simulink model "IF_Flux_Romberg"  (R2022a)
settings: Solver=FixedStepDiscrete  StartTime=0.0  StopTime=3  FixedStep=0.000001  RelTol=1e-4  EnableMultiTasking=on
InitFcn:
  | Ld=5.25e-3;
  | Lq=12e-3;
  | R=0.958;
  | f=0.1827;
model workspace (MAT data in the model file):
  f = Simulink.Signal
  f.DataType = 'single'
  f.Dimensions = 1
  f.DimensionsMode = 'auto'
  f.Complexity = 'real'
  f.SampleTime = -1
  f.SamplingMode = 'auto'
  f.InitialValue = '0.1827'
values from neighbouring files (symbols this model uses):
  ki_c = 1476    [initialize.m]
  ki_pll = 900    [initialize.m]
  ki_sp = 0.5    [initialize.m]
  kp_c = 3.44    [initialize.m]
  kp_pll = 60    [initialize.m]
  kp_sp = 0.01    [initialize.m]
  L = 0.0014    [initialize.m]
  L1 = -5500    [initialize.m]
  L2 = 68500    [initialize.m]
  Rs = 0.6    [initialize.m]
  Ts = 0.0001    [initialize.m]
undefined symbols (not defined in the file or in its folder): DiscIntNeverNeededParam
libraries: slpidlib x6, mcbcontrolslib x5, eeGeneralControl x3, simulink x2, spsDCVoltageSourceLib x1, spsPermanentMagnetSynchronousMachineLib x1, spsUniversalBridgeLib x1, spspowerguiLib x1
settings Model: Creator=张豪  LastModifiedBy=EE
settings SolverCC: AutoInsertRateTranBlk=on
settings OptimizationCC: DefaultParameterBehavior=Inlined  UseDivisionForNetSlopeComputation=on  GainParamInheritBuiltInType=on  UseFloatMulNetSlope=on  InlineInvariantSignals=on  PassReuseOutputArgsAs=Individual arguments  ZeroExternalMemoryAtStartup=off  ZeroInternalMemoryAtStartup=off  NoFixptDivByZeroProtection=on  EfficientFloat2IntCast=on  LifeSpan=1  OptimizeBlockOrder=speed  DifferentSizesBufferReuse=on  EfficientTunableParamExpr=on
settings DebuggingCC: ParameterTunabilityLossMsg=error  UnconnectedInputMsg=warning  UnconnectedOutputMsg=warning  UnconnectedLineMsg=warning
settings HardwareCC: ProdLongLongMode=on
settings SFSimCC: MATLABDynamicMemAlloc=off
settings RTWCC: SystemTargetFile=ert.tlc  GenCodeOnly=on  TemplateMakefile=ert_default_tmf  DLArmComputeVersion=19.05
settings CodeAppCC: ForceParamTrailComments=on  IgnoreCustomStorageClasses=off  OperatorAnnotations=on  SimulinkDataObjDesc=on  SFDataObjDesc=on  CustomSymbolStrGlobalVar=rt$N$M  CustomSymbolStrType=$N$M  CustomSymbolStrFcn=$N$M$F  CustomSymbolStrMacro=$N$M  InsertBlockDesc=on
settings ERTTargetCC: TargetLangStandard=C99 (ISO)  GenerateSampleERTMain=on  IncludeMdlTerminateFcn=off  CombineSignalStateStructs=on  SupportComplex=off  SupportNonInlinedSFcns=on  InlinedParameterPlacement=NonHierarchical  ERTCustomFileTemplate=example_file_process.tlc  ERTFilePackagingFormat=CompactWithDataFile

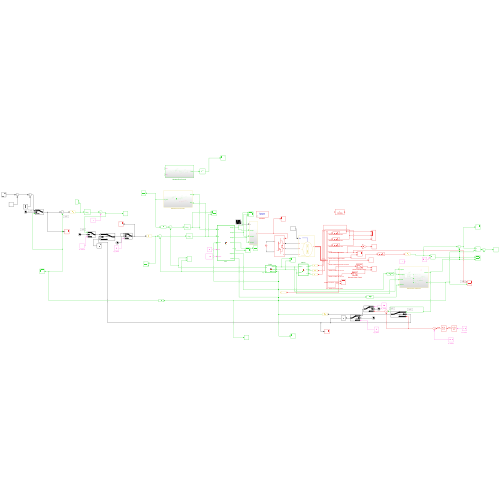
[thumbnail: Simulink's stored preview of the top-level diagram]
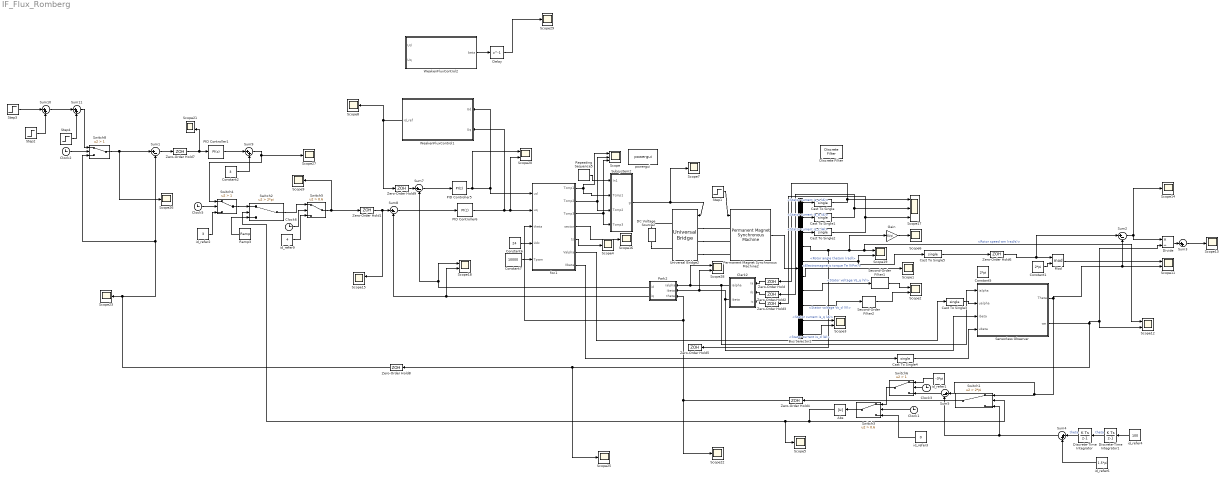
== system IF_Flux_Romberg ==
  Abs : Abs  SaturateOnIntegerOverflow=off
  Bus Selector2 : BusSelector  OutputSignals=Stator current is_a (A),Stator current is_b (A),Stator current is_c (A),Rotor speed wm (rad/s),Rotor angle thetam (rad),Electromagnetic torque Te (N*m),Stator voltage Vs_q (V),Stator voltage Vs_d (V),Stator current is_q (A),Stator current is_d (A)
  Cast To Single{,1..5} (6 alike) : DataTypeConversion  OutDataTypeStr=single  SaturateOnIntegerOverflow=off  RndMeth=Floor
  Clark2 : MATLAB Function  TreatAsAtomicUnit=on
  Clock{1..3,5..6} (5 alike) : Clock
  Constant1 : Constant  Value=2*pi  OutDataTypeStr=single
  Constant2 : Constant  Value=3
  Constant5 : Constant  Value=2*pi  OutDataTypeStr=single
  Constant6 : Constant  Value=24
  Constant7 : Constant  Value=10000  OutDataTypeStr=single
  DC Voltage Source2 : spsDCVoltageSourceLib/DC Voltage Source  Amplitude=24  Measurements=None
  Delay : Delay  DelayLength=1  InitialCondition=0
  Discrete Filter : DiscreteFilter  FilterStructure=Direct form I
  Discrete-Time Integrator : DiscreteIntegrator  SampleTime=-1  ICPrevOutput=DiscIntNeverNeededParam  ICPrevScaledInput=DiscIntNeverNeededParam
  Discrete-Time Integrator1 : DiscreteIntegrator  SampleTime=-1  ICPrevOutput=DiscIntNeverNeededParam  ICPrevScaledInput=DiscIntNeverNeededParam
  Divide : Product  Inputs=*/
  Gain : Gain  Gain=30/pi
  Mod : Math  Operator=mod
  PID Controller1 : slpidlib/PID Controller  Controller=PI  Form=Parallel  TimeDomain=Discrete-time  UseExternalTs=off  SampleTime=1e-4  IntegratorMethod=Forward Euler  FilterMethod=Forward Euler  ControllerParametersSource=internal  P=kp_sp  I=ki_sp  UseKiTs=off  D=0  N=100  UseFilter=on  TunerSelectOption=Transfer Function Based (PID Tuner App)  InitialConditionSource=internal  InitialConditionForIntegrator=0  InitialConditionForFilter=0  DifferentiatorICPrevScaledInput=0  ExternalReset=none  TrackingMode=off  Kt=1  LimitOutput=off  SatLimitsSource=internal  UpperSaturationLimit=7  LowerSaturationLimit=-7  LinearizeAsGain=on  AntiWindupMode=none  Kb=1  POutMin=[]  POutMax=[]  IOutMin=[]  IOutMax=[]  DOutMin=[]  DOutMax=[]  NOutMin=[]  NOutMax=[]  SumOutMin=[]  SumOutMax=[]  SaturationOutMin=[]  SaturationOutMax=[]  PParamMin=[]  PParamMax=[]  IParamMin=[]  IParamMax=[]  DParamMin=[]  DParamMax=[]  NParamMin=[]  NParamMax=[]  KbParamMin=[]  KbParamMax=[]  KtParamMin=[]  KtParamMax=[]  KbOutMin=[]  KbOutMax=[]  KtOutMin=[]  KtOutMax=[]  IntegratorOutMin=[]  IntegratorOutMax=[]  FilterOutMin=[]  FilterOutMax=[]  SumI1OutMin=[]  SumI1OutMax=[]  SumI2OutMin=[]  SumI2OutMax=[]  SumI3OutMin=[]  SumI3OutMax=[]  SumI4OutMin=[]  SumI4OutMax=[]  SumDOutMin=[]  SumDOutMax=[]  DifferentiatorOutMin=[]  DifferentiatorOutMax=[]  FilterDiffOutCoefMin=[]  FilterDiffOutCoefMax=[]  ReciprocalOutMin=[]  ReciprocalOutMax=[]  SumDenOutMin=[]  SumDenOutMax=[]  SumNumOutMin=[]  SumNumOutMax=[]  DivideOutMin=[]  DivideOutMax=[]  UdiffTsProdOutMin=[]  UdiffTsProdOutMax=[]  NTsProdOutMin=[]  NTsProdOutMax=[]  UintegralTsProdOutMin=[]  UintegralTsProdOutMax=[]  UngainTsProdOutMin=[]  UngainTsProdOutMax=[]  IntegratorContinuousStateAttributes=''  IntegratorStateMustResolveToSignalObject=off  IntegratorRTWStateStorageClass=Auto  FilterContinuousStateAttributes=''  FilterStateMustResolveToSignalObject=off  FilterRTWStateStorageClass=Auto  ParallelPVariant=InternalParameters  IdealPVariant=Disabled  IVariant=InternalParameters  DVariant=Disabled  IntegratorVariant=Discrete  SatVariant=Disabled  AWVariant=Passthrough  PCopyVariant=Disabled  TRVariant=Disabled  FdbkBlocksVariant=Forward  IdealPFdbkVariant=Disabled  SatFdbkVariant=Disabled  DerivativeFilterVariant=Disabled  NVariant=Disabled  NCopyVariant=Disabled_SignalSpec  FilterICVariant=Disabled  IntegratorICVariant=InternalICs  ExternalResetVariant=Disabled  TRSumVariant=Passthrough  SumFdbkVariant=Disabled  SumVariant=Sum_PI  TsampFilterVariant=InternalTs  TsampNgainVariant=Passthrough  TsampIntegralVariant=Passthrough  ExternalSaturationOutDataTypeStr=Inherit: Same as second input  aMode=0
  PID Controller5 : slpidlib/PID Controller  Controller=PI  Form=Parallel  TimeDomain=Discrete-time  UseExternalTs=off  SampleTime=1e-4  IntegratorMethod=Forward Euler  FilterMethod=Forward Euler  ControllerParametersSource=internal  P=kp_c  I=ki_c  UseKiTs=off  D=0  N=100  UseFilter=on  TunerSelectOption=Transfer Function Based (PID Tuner App)  InitialConditionSource=internal  InitialConditionForIntegrator=0  InitialConditionForFilter=0  DifferentiatorICPrevScaledInput=0  ExternalReset=none  TrackingMode=off  Kt=1  LimitOutput=off  SatLimitsSource=internal  UpperSaturationLimit=13  LowerSaturationLimit=-10  LinearizeAsGain=on  AntiWindupMode=none  Kb=1  POutMin=[]  POutMax=[]  IOutMin=[]  IOutMax=[]  DOutMin=[]  DOutMax=[]  NOutMin=[]  NOutMax=[]  SumOutMin=[]  SumOutMax=[]  SaturationOutMin=[]  SaturationOutMax=[]  PParamMin=[]  PParamMax=[]  IParamMin=[]  IParamMax=[]  DParamMin=[]  DParamMax=[]  NParamMin=[]  NParamMax=[]  KbParamMin=[]  KbParamMax=[]  KtParamMin=[]  KtParamMax=[]  KbOutMin=[]  KbOutMax=[]  KtOutMin=[]  KtOutMax=[]  IntegratorOutMin=[]  IntegratorOutMax=[]  FilterOutMin=[]  FilterOutMax=[]  SumI1OutMin=[]  SumI1OutMax=[]  SumI2OutMin=[]  SumI2OutMax=[]  SumI3OutMin=[]  SumI3OutMax=[]  SumI4OutMin=[]  SumI4OutMax=[]  SumDOutMin=[]  SumDOutMax=[]  DifferentiatorOutMin=[]  DifferentiatorOutMax=[]  FilterDiffOutCoefMin=[]  FilterDiffOutCoefMax=[]  ReciprocalOutMin=[]  ReciprocalOutMax=[]  SumDenOutMin=[]  SumDenOutMax=[]  SumNumOutMin=[]  SumNumOutMax=[]  DivideOutMin=[]  DivideOutMax=[]  UdiffTsProdOutMin=[]  UdiffTsProdOutMax=[]  NTsProdOutMin=[]  NTsProdOutMax=[]  UintegralTsProdOutMin=[]  UintegralTsProdOutMax=[]  UngainTsProdOutMin=[]  UngainTsProdOutMax=[]  IntegratorContinuousStateAttributes=''  IntegratorStateMustResolveToSignalObject=off  IntegratorRTWStateStorageClass=Auto  FilterContinuousStateAttributes=''  FilterStateMustResolveToSignalObject=off  FilterRTWStateStorageClass=Auto  ParallelPVariant=InternalParameters  IdealPVariant=Disabled  IVariant=InternalParameters  DVariant=Disabled  IntegratorVariant=Discrete  SatVariant=Disabled  AWVariant=Passthrough  PCopyVariant=Disabled  TRVariant=Disabled  FdbkBlocksVariant=Forward  IdealPFdbkVariant=Disabled  SatFdbkVariant=Disabled  DerivativeFilterVariant=Disabled  NVariant=Disabled  NCopyVariant=Disabled_SignalSpec  FilterICVariant=Disabled  IntegratorICVariant=InternalICs  ExternalResetVariant=Disabled  TRSumVariant=Passthrough  SumFdbkVariant=Disabled  SumVariant=Sum_PI  TsampFilterVariant=InternalTs  TsampNgainVariant=Passthrough  TsampIntegralVariant=Passthrough  ExternalSaturationOutDataTypeStr=Inherit: Same as second input  aMode=0
  PID Controller6 : slpidlib/PID Controller  Controller=PI  Form=Parallel  TimeDomain=Discrete-time  UseExternalTs=off  SampleTime=1e-4  IntegratorMethod=Forward Euler  FilterMethod=Forward Euler  ControllerParametersSource=internal  P=kp_c  I=ki_c  UseKiTs=off  D=0  N=100  UseFilter=on  TunerSelectOption=Transfer Function Based (PID Tuner App)  InitialConditionSource=internal  InitialConditionForIntegrator=0  InitialConditionForFilter=0  DifferentiatorICPrevScaledInput=0  ExternalReset=none  TrackingMode=off  Kt=1  LimitOutput=off  SatLimitsSource=internal  UpperSaturationLimit=14  LowerSaturationLimit=0  LinearizeAsGain=on  AntiWindupMode=none  Kb=1  POutMin=[]  POutMax=[]  IOutMin=[]  IOutMax=[]  DOutMin=[]  DOutMax=[]  NOutMin=[]  NOutMax=[]  SumOutMin=[]  SumOutMax=[]  SaturationOutMin=[]  SaturationOutMax=[]  PParamMin=[]  PParamMax=[]  IParamMin=[]  IParamMax=[]  DParamMin=[]  DParamMax=[]  NParamMin=[]  NParamMax=[]  KbParamMin=[]  KbParamMax=[]  KtParamMin=[]  KtParamMax=[]  KbOutMin=[]  KbOutMax=[]  KtOutMin=[]  KtOutMax=[]  IntegratorOutMin=[]  IntegratorOutMax=[]  FilterOutMin=[]  FilterOutMax=[]  SumI1OutMin=[]  SumI1OutMax=[]  SumI2OutMin=[]  SumI2OutMax=[]  SumI3OutMin=[]  SumI3OutMax=[]  SumI4OutMin=[]  SumI4OutMax=[]  SumDOutMin=[]  SumDOutMax=[]  DifferentiatorOutMin=[]  DifferentiatorOutMax=[]  FilterDiffOutCoefMin=[]  FilterDiffOutCoefMax=[]  ReciprocalOutMin=[]  ReciprocalOutMax=[]  SumDenOutMin=[]  SumDenOutMax=[]  SumNumOutMin=[]  SumNumOutMax=[]  DivideOutMin=[]  DivideOutMax=[]  UdiffTsProdOutMin=[]  UdiffTsProdOutMax=[]  NTsProdOutMin=[]  NTsProdOutMax=[]  UintegralTsProdOutMin=[]  UintegralTsProdOutMax=[]  UngainTsProdOutMin=[]  UngainTsProdOutMax=[]  IntegratorContinuousStateAttributes=''  IntegratorStateMustResolveToSignalObject=off  IntegratorRTWStateStorageClass=Auto  FilterContinuousStateAttributes=''  FilterStateMustResolveToSignalObject=off  FilterRTWStateStorageClass=Auto  ParallelPVariant=InternalParameters  IdealPVariant=Disabled  IVariant=InternalParameters  DVariant=Disabled  IntegratorVariant=Discrete  SatVariant=Disabled  AWVariant=Passthrough  PCopyVariant=Disabled  TRVariant=Disabled  FdbkBlocksVariant=Forward  IdealPFdbkVariant=Disabled  SatFdbkVariant=Disabled  DerivativeFilterVariant=Disabled  NVariant=Disabled  NCopyVariant=Disabled_SignalSpec  FilterICVariant=Disabled  IntegratorICVariant=InternalICs  ExternalResetVariant=Disabled  TRSumVariant=Passthrough  SumFdbkVariant=Disabled  SumVariant=Sum_PI  TsampFilterVariant=InternalTs  TsampNgainVariant=Passthrough  TsampIntegralVariant=Passthrough  ExternalSaturationOutDataTypeStr=Inherit: Same as second input  aMode=0
  Park2 : MATLAB Function  TreatAsAtomicUnit=on
  Permanent Magnet Synchronous Machine2 : spsPermanentMagnetSynchronousMachineLib/Permanent Magnet Synchronous Machine  NbPhases=3  FluxDistribution=Sinusoidal  RotorType=Round  MechanicalLoad=Torque Tm  PresetModel=No  ShowDetailedParameters=on  MeasurementBus=off  Resistance=0.6  Inductance=8.5e-3  dqInductances=[5.25e-3 12e-3]  La=1.4e-3  MachineConstant=Flux linkage established by magnets (V.s)  Flux=0.034182  VoltageCst=6.1999  TorqueCst=0.051273  Flat=120  Mechanical=[1.1e-5 0.001 1 0.02]  PolePairs=4  InitialConditions=[0,0, 0,0]  InitialConditions5ph=[0 0 0 0 0 0]  RefAngle=Aligned with phase A axis (original Park)  IterativeDiscreteModel=Trapezoidal non iterative  TsBlock=-1  TsPowergui=0
  Ramp3 : simulink/Sources/Ramp  slope=-10  start=0.6  InitialOutput=4
  Repeating Sequence5 : simulink/Sources/Repeating Sequence  rep_seq_t=[0 0.00005 0.0001]  rep_seq_y=[0 5000 0]
  Scope : Scope  NumInputPorts=3
  Scope{1,4..9,13..14,16,22..23,25..27,29} (16 alike) : Scope
  Scope{2..3,11..12,15,18..21,28} (10 alike) : Scope  NumInputPorts=2
  Scope17 : Scope  NumInputPorts=3
  Second-Order Filter1 : eeGeneralControl/Second-Order Filter  FilterType=Low-pass  fn=100  Zeta=1  Ts=-1  A0=0  Ph0=0  f0=0  b0=0
      settings: SourceProductBaseCode=PS
  Second-Order Filter2 : eeGeneralControl/Second-Order Filter  FilterType=Low-pass  fn=100  Zeta=1  Ts=-1  A0=0  Ph0=0  f0=0  b0=0
      settings: SourceProductBaseCode=PS
  Sensorless Observer : Subsystem
  Step1 : Step  Time=0.6  Before=0.05  After=0.05  SampleTime=0
  Step2 : Step  Time=2  After=80  SampleTime=0
  Step3 : Step  Time=1.5  Before=150  After=200  SampleTime=0
  Step4 : Step  Time=2.5  After=-100  SampleTime=0
  Subsystem2 : Subsystem
  Sum{1..2,5,7..8} (5 alike) : Sum  Inputs=|+-
  Sum{3..4,9..11} (5 alike) : Sum  Inputs=|++
  Switch1 : Switch  Criteria=u2 > Threshold  Threshold=2*pi  SaturateOnIntegerOverflow=off  InputSameDT=off
  Switch2 : Switch  Criteria=u2 > Threshold  Threshold=2*pi  SaturateOnIntegerOverflow=off  InputSameDT=off
  Switch3 : Switch  Criteria=u2 > Threshold  Threshold=0.6  SaturateOnIntegerOverflow=off  InputSameDT=off
  Switch4 : Switch  Criteria=u2 > Threshold  Threshold=1  SaturateOnIntegerOverflow=off  InputSameDT=off
  Switch5 : Switch  Criteria=u2 > Threshold  Threshold=0.6  SaturateOnIntegerOverflow=off  InputSameDT=off
  Switch6 : Switch  Criteria=u2 > Threshold  Threshold=1  SaturateOnIntegerOverflow=off  InputSameDT=off
  Switch8 : Switch  Criteria=u2 > Threshold  Threshold=1  SaturateOnIntegerOverflow=off  InputSameDT=off
  Universal Bridge2 : spsUniversalBridgeLib/Universal Bridge  Arms=3  SnubberResistance=1e5  SnubberCapacitance=inf  Device=IGBT / Diodes  Ron=1e-3  Lon=0  ForwardVoltages="[  0  0  ]"  ForwardVoltage=0  GTOparameters=[ 10e-6 , 20e-6 ]  IGBTparameters=[ 1e-6 , 2e-6 ]  Measurements=None  Measurements_2=None  converterType=Rectifier
  WeakenFluxControl1 : Subsystem
  WeakenFluxControl2 : Subsystem
  Zero-Order Hold{,1..9} (10 alike) : ZeroOrderHold  SampleTime=1e-4
  foc1 : MATLAB Function  TreatAsAtomicUnit=on
  id_refer1 : Constant  Value=-3*pi
  id_refer2 : Constant  Value=3
  id_refer3 : Constant  Value=0
  id_refer4 : Constant  Value=100
  id_refer6 : Constant  Value=1.5*pi
  id_refer9 : Constant  Value=4
  powergui : spspowerguiLib/powergui  Priority=1  SimulationMode=Discrete  SampleTime=1e-6  frequency=60  Iterations=50  frequencyindice=0  Pbase=100e6  ErrMax=1e-4  UnitsV=kV  UnitsW=MW  buscounter=0  FunctionMessages=off  echomessages=off  EnableUseOfTLC=off  CurrentSourceSwitches=off  DisableSnubberDevices=off  DisableRonSwitches=off  DisableVfSwitches=off  DisplayEquations=off  AutomaticDiscreteSolvers=off  SolverType=Tustin/Backward Euler (TBE)  Interpol=off  ExternalGateDelay=off  methode=off  Ts=100  x0status=blocks  SPID=on  SwTol=0  HookPort=off  NonlinearTolerance=1e-4  nMaxIteration=100  ContinueOnMaxIteration=off  RestoreLinks=warning  ResistiveCurrentMeasurement=off  Frange=[0:2:500]  Ylog=off  Xlog=on  ShowGrid=off  save=off  variable=ZData  structure=0  ZoomFFT=off  StartTime=0.0  cycles=1  DisplayStyle=1  fundamental=60  FreqAxis=off  MaxFrequency=1000  frequencyindicesteady=1  RmsSteady=1  display=off
  wires:
  Repeating Sequence5/1 -> Subsystem2/1(In1)
  Constant7/1 -> foc1/5(Tpwm)
  foc1/3(Tcmp3) -> Subsystem2/4(Tcmp3), Scope/3
  foc1/2(Tcmp2) -> Subsystem2/3(Tcmp2), Scope/2
  Constant6/1 -> foc1/4(Udc)
  foc1/1(Tcmp1) -> Subsystem2/2(Tcmp1), Scope/1
  foc1/4(sector) -> Scope16/1
  Subsystem2/1(g) -> Scope7/1, Universal Bridge2/1
  Permanent Magnet Synchronous Machine2/1 -> Bus Selector2/1
  Bus Selector2/1 -> Cast To Single/1  "<Stator current is_a (A)>"
  Bus Selector2/2 -> Cast To Single1/1  "<Stator current is_b (A)>"
  Bus Selector2/3 -> Cast To Single2/1  "<Stator current is_c (A)>"
  Bus Selector2/5 -> Scope19/2, Cast To Single5/1  "<Rotor angle thetam (rad)>"
  Bus Selector2/4 -> Scope12/1, Scope19/1, Gain/1, Zero-Order Hold5/1  "<Rotor speed wm (rad/s)>"
  Bus Selector2/6 -> Scope1/1  "<Electromagnetic torque Te (N*m)>"
  Bus Selector2/7 -> Second-Order Filter1/1  "<Stator voltage Vs_q (V)>"
  Bus Selector2/8 -> Second-Order Filter2/1  "<Stator voltage Vs_d (V)>"
  Second-Order Filter1/1 -> Scope2/1
  Second-Order Filter2/1 -> Scope2/2
  Bus Selector2/9 -> Scope3/1  "<Stator current is_q (A)>"
  Bus Selector2/10 -> Scope3/2  "<Stator current is_d (A)>"
  foc1/5(ts) -> Scope4/1
  Gain/1 -> Scope6/1
  Zero-Order Hold/1 -> Clark2/1(ia)
  Zero-Order Hold2/1 -> Clark2/2(ib)
  Zero-Order Hold3/1 -> Clark2/3(ic)
  Zero-Order Hold4/1 -> foc1/3(theta), Park2/3(theta), Scope22/1
  Sum8/1 -> PID Controller6/1
  Step1/1 -> Permanent Magnet Synchronous Machine2/1
  Cast To Single/1 -> Zero-Order Hold/1, Scope17/1
  Cast To Single1/1 -> Zero-Order Hold2/1, Scope17/2
  Cast To Single2/1 -> Zero-Order Hold3/1, Scope17/3
  foc1/6(Valpha) -> Cast To Single3/1
  foc1/7(Vbeta) -> Cast To Single4/1
  Cast To Single3/1 -> Sensorless Observer/2(ualpha)
  Cast To Single4/1 -> Sensorless Observer/4(ubeta)
  Cast To Single5/1 -> Zero-Order Hold6/1
  Constant1/1 -> Mod/2
  Zero-Order Hold6/1 -> Sum2/1, Mod/1
  Sum2/1 -> Divide/1, Scope14/1
  Divide/1 -> Sum3/1
  Sum3/1 -> Scope13/1
  Zero-Order Hold1/1 -> Scope15/1, Sum8/1
  Switch8/1 -> Sum1/1, Scope26/1
  Discrete-Time Integrator1/1 -> Discrete-Time Integrator/1  "theta"
  Discrete-Time Integrator/1 -> Sum4/1  "theta"
  id_refer4/1 -> Discrete-Time Integrator1/1
  id_refer6/1 -> Sum4/2
  id_refer9/1 -> Switch5/3
  Clock6/1 -> Switch5/2
  Sum7/1 -> PID Controller5/1
  Sum4/1 -> Sum5/2, Switch1/3
  Zero-Order Hold8/1 -> Switch8/3, Sum1/2, Scope23/1
  Ramp3/1 -> Switch2/3
  Switch2/1 -> Switch5/1
  Switch3/1 -> Abs/1
  id_refer3/1 -> Switch3/3
  Clock1/1 -> Switch3/2
  Zero-Order Hold7/1 -> Scope21/2, PID Controller1/1
  Clock2/1 -> Switch8/2
  Clock5/1 -> Switch4/2
  id_refer2/1 -> Switch4/3
  Sensorless Observer/1(Theta) -> Scope11/2, Sum2/2, Switch1/1, Sum5/1
  Abs/1 -> Scope5/1, Switch2/2, Switch1/2
  Zero-Order Hold9/1 -> Sum7/1
  Constant2/1 -> Sum9/2
  Sum1/1 -> Zero-Order Hold7/1
  PID Controller1/1 -> Sum9/1
  Sum9/1 -> Scope27/1, Switch4/1
  Step3/1 -> Sum10/1
  Switch4/1 -> Switch2/1
  Clark2/1(ialpha) -> Sensorless Observer/1(ialpha), Scope28/1, Park2/1(ialpha)
  Clark2/2(ibeta) -> Sensorless Observer/3(ibeta), Scope28/2, Park2/2(ibeta)
  Sensorless Observer/2(we) -> Divide/2, Scope12/2, Zero-Order Hold8/1, Scope25/1
  Step2/1 -> Sum10/2
  Sum10/1 -> Sum11/1
  Sum11/1 -> Switch8/1
  Step4/1 -> Sum11/2
  Mod/1 -> Scope11/1
  WeakenFluxControl1/1(id_ref) -> Scope8/1, Zero-Order Hold9/1
  Park2/2(iq) -> Scope18/2, Sum8/2
  Park2/1(id) -> Scope18/1, Sum7/2
  PID Controller6/1 -> foc1/2(uq), Scope20/2, WeakenFluxControl1/2(Uq)
  PID Controller5/1 -> WeakenFluxControl1/1(Ud), foc1/1(ud), Scope20/1
  Switch1/1 -> Zero-Order Hold4/1
  Sum5/1 -> Switch6/3
  Clock3/1 -> Switch6/2
  id_refer1/1 -> Switch6/1
  Switch6/1 -> Switch3/1
  Delay/1 -> Scope29/1
  WeakenFluxControl2/1(beta) -> Delay/1
  Switch5/1 -> Scope9/1, Zero-Order Hold1/1
  connections:
  DC Voltage Source2/LConn1 -- Universal Bridge2/RConn2
  DC Voltage Source2/RConn1 -- Universal Bridge2/RConn1
  Universal Bridge2/LConn1 -- Permanent Magnet Synchronous Machine2/LConn1
  Universal Bridge2/LConn3 -- Permanent Magnet Synchronous Machine2/LConn3
  Universal Bridge2/LConn2 -- Permanent Magnet Synchronous Machine2/LConn2

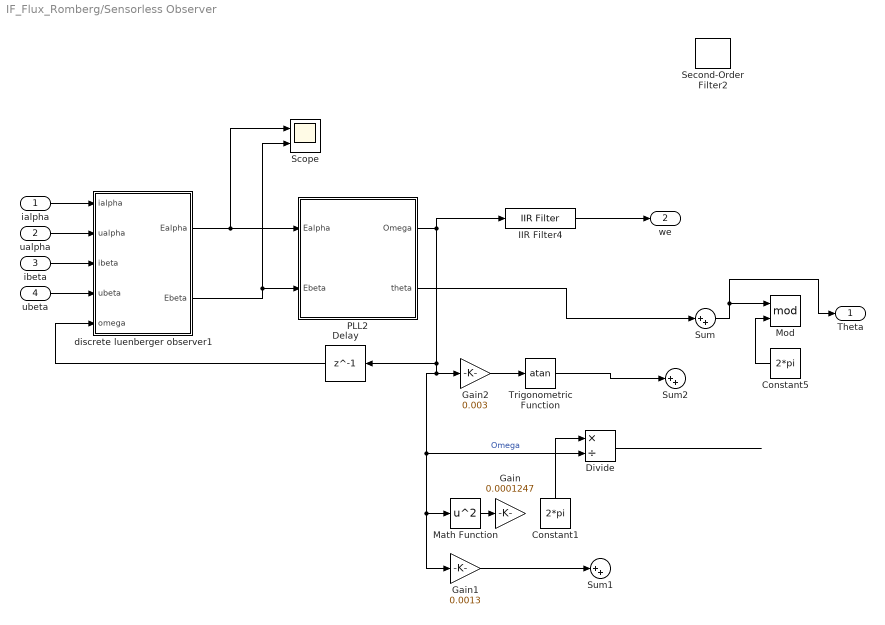
== system IF_Flux_Romberg/Sensorless Observer ==
  ialpha : Inport  OutDataTypeStr=single
  ualpha : Inport  Port=2  OutDataTypeStr=single
  ibeta : Inport  Port=3  OutDataTypeStr=single
  ubeta : Inport  Port=4  OutDataTypeStr=single
  Constant1 : Constant  Value=2*pi  OutDataTypeStr=single
  Constant5 : Constant  Value=2*pi  OutDataTypeStr=single
  Delay : Delay  DelayLength=1  InputProcessing=Columns as channels (frame based)
  Divide : Product  Inputs=*/
  Gain : Gain  Gain=0.0001247
  Gain1 : Gain  Gain=0.0013
  Gain2 : Gain  Gain=0.003
  IIR Filter4 : mcbcontrolslib/IIR Filter  VariantControl=Low Pass Filter  VariantSelect=Low-pass  Filter_constant=0.01  advancedSettings=on  Ts=1e-4  cutOff_freq=16.0763
      settings: SourceProductBaseCode=MT
  Math Function : Math  Operator=square
  Mod : Math  Operator=mod
  PLL2 : Subsystem
  Scope : Scope  NumInputPorts=2
  Second-Order Filter2 : eeGeneralControl/Second-Order Filter  FilterType=Low-pass  fn=100  Zeta=1  Ts=-1  A0=0  Ph0=0  f0=0  b0=0
      settings: SourceProductBaseCode=PS
  Sum : Sum  Inputs=|++
  Sum1 : Sum  Inputs=|++
  Sum2 : Sum  Inputs=|++
  Trigonometric Function : Trigonometry  Operator=atan
  discrete luenberger observer1 : Subsystem
  Theta : Outport
  we : Outport  Port=2
  wires:
  ubeta/1 -> discrete luenberger observer1/4(ubeta)
  ualpha/1 -> discrete luenberger observer1/2(ualpha)
  ibeta/1 -> discrete luenberger observer1/3(ibeta)
  ialpha/1 -> discrete luenberger observer1/1(ialpha)
  discrete luenberger observer1/1(Ealpha) -> Scope/1, PLL2/1(Ealpha)
  discrete luenberger observer1/2(Ebeta) -> Scope/2, PLL2/2(Ebeta)
  Constant5/1 -> Mod/2
  Delay/1 -> discrete luenberger observer1/5(omega)
  PLL2/2(theta) -> Sum/1
  Sum/1 -> Theta/1, Mod/1
  Math Function/1 -> Gain/1
  PLL2/1(Omega) -> IIR Filter4/1, Delay/1, Gain1/1, Math Function/1, Divide/2, Gain2/1  "Omega"
  Gain1/1 -> Sum1/1
  Constant1/1 -> Divide/1
  Gain2/1 -> Trigonometric Function/1
  Trigonometric Function/1 -> Sum2/1
  IIR Filter4/1 -> we/1
  Divide/1 -> ?

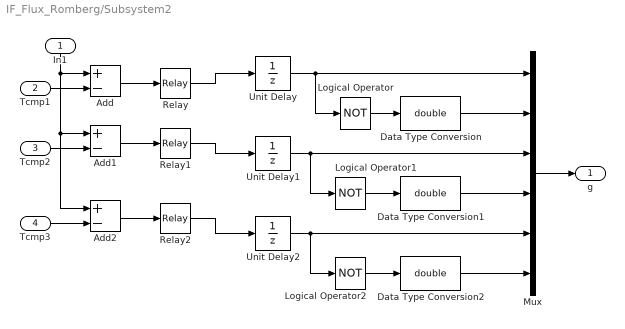
== system IF_Flux_Romberg/Subsystem2 ==
  In1 : Inport
  Tcmp1 : Inport  Port=2
  Tcmp2 : Inport  Port=3
  Tcmp3 : Inport  Port=4
  Add : Sum  Inputs=+-
  Add1 : Sum  Inputs=+-
  Add2 : Sum  Inputs=+-
  Data Type Conversion : DataTypeConversion  OutDataTypeStr=double  SaturateOnIntegerOverflow=off  RndMeth=Floor
  Data Type Conversion1 : DataTypeConversion  OutDataTypeStr=double  SaturateOnIntegerOverflow=off  RndMeth=Floor
  Data Type Conversion2 : DataTypeConversion  OutDataTypeStr=double  SaturateOnIntegerOverflow=off  RndMeth=Floor
  Logical Operator : Logic  Operator=NOT  AllPortsSameDT=off  OutDataTypeStr=boolean
  Logical Operator1 : Logic  Operator=NOT  AllPortsSameDT=off  OutDataTypeStr=boolean
  Logical Operator2 : Logic  Operator=NOT  AllPortsSameDT=off  OutDataTypeStr=boolean
  Mux : Mux  Inputs=6
  Relay : Relay  OffSwitchValue=-eps
  Relay1 : Relay  OffSwitchValue=-eps
  Relay2 : Relay  OffSwitchValue=-eps
  Unit Delay : UnitDelay  SampleTime=-1  HasFrameUpgradeWarning=on
  Unit Delay1 : UnitDelay  SampleTime=-1  HasFrameUpgradeWarning=on
  Unit Delay2 : UnitDelay  SampleTime=-1  HasFrameUpgradeWarning=on
  g : Outport  VectorParamsAs1DForOutWhenUnconnected=off
  wires:
  Tcmp3/1 -> Add2/2
  Tcmp2/1 -> Add1/2
  Tcmp1/1 -> Add/2
  Relay2/1 -> Unit Delay2/1
  Relay1/1 -> Unit Delay1/1
  Relay/1 -> Unit Delay/1
  Unit Delay2/1 -> Mux/5, Logical Operator2/1
  Unit Delay1/1 -> Mux/3, Logical Operator1/1
  Unit Delay/1 -> Logical Operator/1, Mux/1
  Mux/1 -> g/1
  Data Type Conversion/1 -> Mux/2
  Data Type Conversion1/1 -> Mux/4
  Data Type Conversion2/1 -> Mux/6
  Logical Operator2/1 -> Data Type Conversion2/1
  Logical Operator1/1 -> Data Type Conversion1/1
  Logical Operator/1 -> Data Type Conversion/1
  Add1/1 -> Relay1/1
  Add2/1 -> Relay2/1
  Add/1 -> Relay/1
  In1/1 -> Add/1, Add2/1, Add1/1

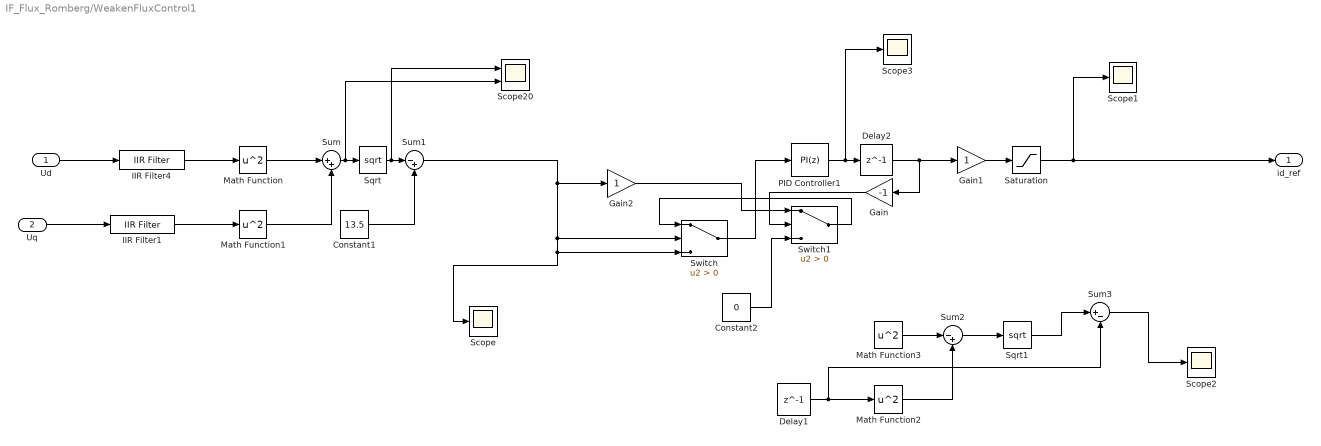
== system IF_Flux_Romberg/WeakenFluxControl1 ==
  Ud : Inport  OutDataTypeStr=double
  Uq : Inport  Port=2  OutDataTypeStr=double
  Constant1 : Constant  Value=13.5
  Constant2 : Constant  Value=0
  Delay1 : Delay  DelayLength=1  InitialCondition=0
  Delay2 : Delay  DelayLength=1  InitialCondition=0
  Gain : Gain  Gain=-1
  Gain1 : Gain
  Gain2 : Gain
  IIR Filter1 : mcbcontrolslib/IIR Filter  VariantControl=Low Pass Filter  VariantSelect=Low-pass  Filter_constant=0.05  advancedSettings=on  Ts=1e-4  cutOff_freq=83.7658
      settings: SourceProductBaseCode=MT
  IIR Filter4 : mcbcontrolslib/IIR Filter  VariantControl=Low Pass Filter  VariantSelect=Low-pass  Filter_constant=0.05  advancedSettings=on  Ts=1e-4  cutOff_freq=83.7658
      settings: SourceProductBaseCode=MT
  Math Function{,1..3} (4 alike) : Math  Operator=square
  PID Controller1 : slpidlib/PID Controller  Controller=PI  Form=Parallel  TimeDomain=Discrete-time  UseExternalTs=off  SampleTime=1e-4  IntegratorMethod=Forward Euler  FilterMethod=Forward Euler  ControllerParametersSource=internal  P=1.5  I=10  UseKiTs=off  D=0  N=100  UseFilter=off  TunerSelectOption=Transfer Function Based (PID Tuner App)  InitialConditionSource=internal  InitialConditionForIntegrator=0  InitialConditionForFilter=0  DifferentiatorICPrevScaledInput=0  ExternalReset=none  TrackingMode=off  Kt=1  LimitOutput=on  SatLimitsSource=internal  UpperSaturationLimit=0  LowerSaturationLimit=-10  LinearizeAsGain=on  AntiWindupMode=none  Kb=1  POutMin=[]  POutMax=[]  IOutMin=[]  IOutMax=[]  DOutMin=[]  DOutMax=[]  NOutMin=[]  NOutMax=[]  SumOutMin=[]  SumOutMax=[]  SaturationOutMin=[]  SaturationOutMax=[]  PParamMin=[]  PParamMax=[]  IParamMin=[]  IParamMax=[]  DParamMin=[]  DParamMax=[]  NParamMin=[]  NParamMax=[]  KbParamMin=[]  KbParamMax=[]  KtParamMin=[]  KtParamMax=[]  KbOutMin=[]  KbOutMax=[]  KtOutMin=[]  KtOutMax=[]  IntegratorOutMin=[]  IntegratorOutMax=[]  FilterOutMin=[]  FilterOutMax=[]  SumI1OutMin=[]  SumI1OutMax=[]  SumI2OutMin=[]  SumI2OutMax=[]  SumI3OutMin=[]  SumI3OutMax=[]  SumI4OutMin=[]  SumI4OutMax=[]  SumDOutMin=[]  SumDOutMax=[]  DifferentiatorOutMin=[]  DifferentiatorOutMax=[]  FilterDiffOutCoefMin=[]  FilterDiffOutCoefMax=[]  ReciprocalOutMin=[]  ReciprocalOutMax=[]  SumDenOutMin=[]  SumDenOutMax=[]  SumNumOutMin=[]  SumNumOutMax=[]  DivideOutMin=[]  DivideOutMax=[]  UdiffTsProdOutMin=[]  UdiffTsProdOutMax=[]  NTsProdOutMin=[]  NTsProdOutMax=[]  UintegralTsProdOutMin=[]  UintegralTsProdOutMax=[]  UngainTsProdOutMin=[]  UngainTsProdOutMax=[]  IntegratorContinuousStateAttributes=''  IntegratorStateMustResolveToSignalObject=off  IntegratorRTWStateStorageClass=Auto  FilterContinuousStateAttributes=''  FilterStateMustResolveToSignalObject=off  FilterRTWStateStorageClass=Auto  ParallelPVariant=InternalParameters  IdealPVariant=Disabled  IVariant=InternalParameters  DVariant=Disabled  IntegratorVariant=Discrete  SatVariant=Enabled  AWVariant=Passthrough  PCopyVariant=Disabled  TRVariant=Disabled  FdbkBlocksVariant=Forward  IdealPFdbkVariant=Disabled  SatFdbkVariant=Disabled  DerivativeFilterVariant=Disabled  NVariant=Disabled  NCopyVariant=Disabled_SignalSpec  FilterICVariant=Disabled  IntegratorICVariant=InternalICs  ExternalResetVariant=Disabled  TRSumVariant=Passthrough  SumFdbkVariant=Disabled  SumVariant=Sum_PI  TsampFilterVariant=InternalTs  TsampNgainVariant=Passthrough  TsampIntegralVariant=Passthrough  ExternalSaturationOutDataTypeStr=Inherit: Same as second input  aMode=0
  Saturation : Saturate  UpperLimit=0  LowerLimit=-24
  Scope{,1..3} (4 alike) : Scope
  Scope20 : Scope  NumInputPorts=2
  Sqrt : Sqrt
  Sqrt1 : Sqrt
  Sum : Sum  Inputs=|++
  Sum1 : Sum  Inputs=|-+
  Sum2 : Sum  Inputs=|-+
  Sum3 : Sum  Inputs=|+-
  Switch : Switch  Criteria=u2 > Threshold  SaturateOnIntegerOverflow=off  InputSameDT=off
  Switch1 : Switch  Criteria=u2 > Threshold  SaturateOnIntegerOverflow=off  InputSameDT=off
  id_ref : Outport
  wires:
  Math Function/1 -> Sum/1
  Math Function1/1 -> Sum/2
  Constant1/1 -> Sum1/2
  Sum/1 -> Scope20/2, Sqrt/1
  Sqrt/1 -> Scope20/1, Sum1/1
  Ud/1 -> IIR Filter4/1
  Uq/1 -> IIR Filter1/1
  IIR Filter4/1 -> Math Function/1
  IIR Filter1/1 -> Math Function1/1
  Gain/1 -> Switch1/2
  Constant2/1 -> Switch1/3
  Switch1/1 -> Switch/1
  ? -> Delay1/1
  Delay1/1 -> Sum3/2, Math Function2/1
  Math Function2/1 -> Sum2/2
  Sum2/1 -> Sqrt1/1
  Math Function3/1 -> Sum2/1
  Sqrt1/1 -> Sum3/1
  Sum3/1 -> Scope2/1
  Switch/1 -> PID Controller1/1
  Delay2/1 -> Gain1/1, Gain/1
  Saturation/1 -> Scope1/1, id_ref/1
  PID Controller1/1 -> Scope3/1, Delay2/1
  Sum1/1 -> Scope/1, Switch/3, Switch/2, Gain2/1
  Gain1/1 -> Saturation/1
  Gain2/1 -> Switch1/1

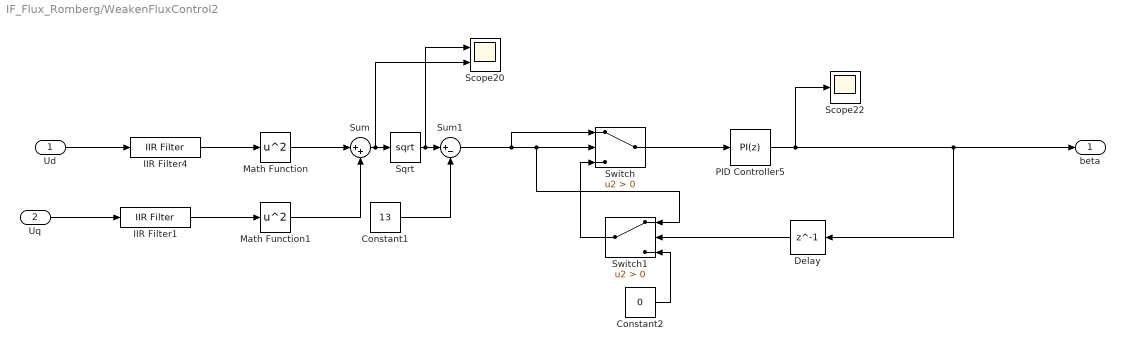
== system IF_Flux_Romberg/WeakenFluxControl2 ==
  Ud : Inport  OutDataTypeStr=double
  Uq : Inport  Port=2  OutDataTypeStr=double
  Constant1 : Constant  Value=13  VectorParams1D=off
  Constant2 : Constant  Value=0  VectorParams1D=off
  Delay : Delay  DelayLength=1  InitialCondition=0
  IIR Filter1 : mcbcontrolslib/IIR Filter  VariantControl=Low Pass Filter  VariantSelect=Low-pass  Filter_constant=0.02  advancedSettings=on  Ts=1e-4  cutOff_freq=32.4806
      settings: SourceProductBaseCode=MT
  IIR Filter4 : mcbcontrolslib/IIR Filter  VariantControl=Low Pass Filter  VariantSelect=Low-pass  Filter_constant=0.02  advancedSettings=on  Ts=1e-4  cutOff_freq=32.4806
      settings: SourceProductBaseCode=MT
  Math Function : Math  Operator=square
  Math Function1 : Math  Operator=square
  PID Controller5 : slpidlib/PID Controller  Controller=PI  Form=Parallel  TimeDomain=Discrete-time  UseExternalTs=off  SampleTime=1e-4  IntegratorMethod=Forward Euler  FilterMethod=Forward Euler  ControllerParametersSource=internal  P=1  I=10  UseKiTs=off  D=0  N=100  UseFilter=on  TunerSelectOption=Transfer Function Based (PID Tuner App)  InitialConditionSource=internal  InitialConditionForIntegrator=0  InitialConditionForFilter=0  DifferentiatorICPrevScaledInput=0  ExternalReset=none  TrackingMode=off  Kt=1  LimitOutput=on  SatLimitsSource=internal  UpperSaturationLimit=1.57  LowerSaturationLimit=0  LinearizeAsGain=on  AntiWindupMode=none  Kb=1  POutMin=[]  POutMax=[]  IOutMin=[]  IOutMax=[]  DOutMin=[]  DOutMax=[]  NOutMin=[]  NOutMax=[]  SumOutMin=[]  SumOutMax=[]  SaturationOutMin=[]  SaturationOutMax=[]  PParamMin=[]  PParamMax=[]  IParamMin=[]  IParamMax=[]  DParamMin=[]  DParamMax=[]  NParamMin=[]  NParamMax=[]  KbParamMin=[]  KbParamMax=[]  KtParamMin=[]  KtParamMax=[]  KbOutMin=[]  KbOutMax=[]  KtOutMin=[]  KtOutMax=[]  IntegratorOutMin=[]  IntegratorOutMax=[]  FilterOutMin=[]  FilterOutMax=[]  SumI1OutMin=[]  SumI1OutMax=[]  SumI2OutMin=[]  SumI2OutMax=[]  SumI3OutMin=[]  SumI3OutMax=[]  SumI4OutMin=[]  SumI4OutMax=[]  SumDOutMin=[]  SumDOutMax=[]  DifferentiatorOutMin=[]  DifferentiatorOutMax=[]  FilterDiffOutCoefMin=[]  FilterDiffOutCoefMax=[]  ReciprocalOutMin=[]  ReciprocalOutMax=[]  SumDenOutMin=[]  SumDenOutMax=[]  SumNumOutMin=[]  SumNumOutMax=[]  DivideOutMin=[]  DivideOutMax=[]  UdiffTsProdOutMin=[]  UdiffTsProdOutMax=[]  NTsProdOutMin=[]  NTsProdOutMax=[]  UintegralTsProdOutMin=[]  UintegralTsProdOutMax=[]  UngainTsProdOutMin=[]  UngainTsProdOutMax=[]  IntegratorContinuousStateAttributes=''  IntegratorStateMustResolveToSignalObject=off  IntegratorRTWStateStorageClass=Auto  FilterContinuousStateAttributes=''  FilterStateMustResolveToSignalObject=off  FilterRTWStateStorageClass=Auto  ParallelPVariant=InternalParameters  IdealPVariant=Disabled  IVariant=InternalParameters  DVariant=Disabled  IntegratorVariant=Discrete  SatVariant=Enabled  AWVariant=Passthrough  PCopyVariant=Disabled  TRVariant=Disabled  FdbkBlocksVariant=Forward  IdealPFdbkVariant=Disabled  SatFdbkVariant=Disabled  DerivativeFilterVariant=Disabled  NVariant=Disabled  NCopyVariant=Disabled_SignalSpec  FilterICVariant=Disabled  IntegratorICVariant=InternalICs  ExternalResetVariant=Disabled  TRSumVariant=Passthrough  SumFdbkVariant=Disabled  SumVariant=Sum_PI  TsampFilterVariant=InternalTs  TsampNgainVariant=Passthrough  TsampIntegralVariant=Passthrough  ExternalSaturationOutDataTypeStr=Inherit: Same as second input  aMode=0
  Scope20 : Scope  NumInputPorts=2
  Scope22 : Scope
  Sqrt : Sqrt
  Sum : Sum  Inputs=|++
  Sum1 : Sum  Inputs=|+-
  Switch : Switch  Criteria=u2 > Threshold  SaturateOnIntegerOverflow=off  InputSameDT=off
  Switch1 : Switch  Criteria=u2 > Threshold  SaturateOnIntegerOverflow=off  InputSameDT=off
  beta : Outport
  wires:
  Math Function/1 -> Sum/1
  Math Function1/1 -> Sum/2
  Sum/1 -> Scope20/2, Sqrt/1
  Sqrt/1 -> Scope20/1, Sum1/1
  Ud/1 -> IIR Filter4/1
  Uq/1 -> IIR Filter1/1
  IIR Filter4/1 -> Math Function/1
  IIR Filter1/1 -> Math Function1/1
  Constant1/1 -> Sum1/2
  PID Controller5/1 -> Scope22/1, Delay/1, beta/1
  Switch/1 -> PID Controller5/1
  Switch1/1 -> Switch/3
  Constant2/1 -> Switch1/3
  Sum1/1 -> Switch/1, Switch1/1, Switch/2
  Delay/1 -> Switch1/2

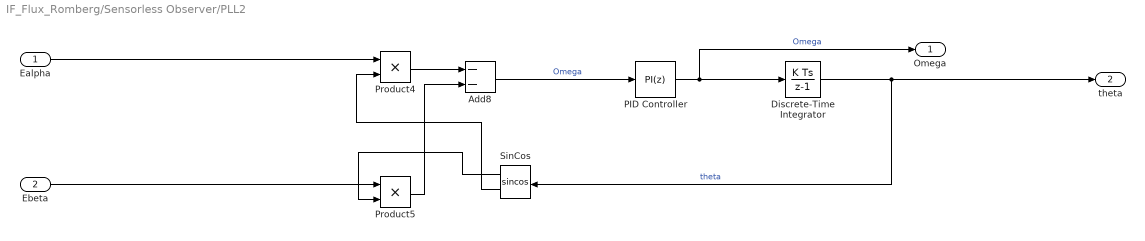
== system IF_Flux_Romberg/Sensorless Observer/PLL2 ==
  Ealpha : Inport
  Ebeta : Inport  Port=2
  Add8 : Sum  Inputs=--
  Discrete-Time Integrator : DiscreteIntegrator  SampleTime=-1  ICPrevOutput=DiscIntNeverNeededParam  ICPrevScaledInput=DiscIntNeverNeededParam
  PID Controller : slpidlib/PID Controller  Controller=PI  Form=Parallel  TimeDomain=Discrete-time  UseExternalTs=off  SampleTime=-1  IntegratorMethod=Forward Euler  FilterMethod=Forward Euler  ControllerParametersSource=internal  P=kp_pll  I=ki_pll  UseKiTs=off  D=0  N=100  UseFilter=on  TunerSelectOption=Transfer Function Based (PID Tuner App)  InitialConditionSource=internal  InitialConditionForIntegrator=0  InitialConditionForFilter=0  DifferentiatorICPrevScaledInput=0  ExternalReset=none  TrackingMode=off  Kt=1  LimitOutput=off  SatLimitsSource=internal  UpperSaturationLimit=2500*2*pi*4/60  LowerSaturationLimit=-2500*2*pi*4/60  LinearizeAsGain=on  AntiWindupMode=clamping  Kb=1  POutMin=[]  POutMax=[]  IOutMin=[]  IOutMax=[]  DOutMin=[]  DOutMax=[]  NOutMin=[]  NOutMax=[]  SumOutMin=[]  SumOutMax=[]  SaturationOutMin=[]  SaturationOutMax=[]  PParamMin=[]  PParamMax=[]  IParamMin=[]  IParamMax=[]  DParamMin=[]  DParamMax=[]  NParamMin=[]  NParamMax=[]  KbParamMin=[]  KbParamMax=[]  KtParamMin=[]  KtParamMax=[]  KbOutMin=[]  KbOutMax=[]  KtOutMin=[]  KtOutMax=[]  IntegratorOutMin=[]  IntegratorOutMax=[]  FilterOutMin=[]  FilterOutMax=[]  SumI1OutMin=[]  SumI1OutMax=[]  SumI2OutMin=[]  SumI2OutMax=[]  SumI3OutMin=[]  SumI3OutMax=[]  SumI4OutMin=[]  SumI4OutMax=[]  SumDOutMin=[]  SumDOutMax=[]  DifferentiatorOutMin=[]  DifferentiatorOutMax=[]  FilterDiffOutCoefMin=[]  FilterDiffOutCoefMax=[]  ReciprocalOutMin=[]  ReciprocalOutMax=[]  SumDenOutMin=[]  SumDenOutMax=[]  SumNumOutMin=[]  SumNumOutMax=[]  DivideOutMin=[]  DivideOutMax=[]  UdiffTsProdOutMin=[]  UdiffTsProdOutMax=[]  NTsProdOutMin=[]  NTsProdOutMax=[]  UintegralTsProdOutMin=[]  UintegralTsProdOutMax=[]  UngainTsProdOutMin=[]  UngainTsProdOutMax=[]  IntegratorContinuousStateAttributes=''  IntegratorStateMustResolveToSignalObject=off  IntegratorRTWStateStorageClass=Auto  FilterContinuousStateAttributes=''  FilterStateMustResolveToSignalObject=off  FilterRTWStateStorageClass=Auto  ParallelPVariant=InternalParameters  IdealPVariant=Disabled  IVariant=InternalParameters  DVariant=Disabled  IntegratorVariant=Discrete  SatVariant=Disabled  AWVariant=Passthrough  PCopyVariant=Disabled  TRVariant=Disabled  FdbkBlocksVariant=Forward  IdealPFdbkVariant=Disabled  SatFdbkVariant=Disabled  DerivativeFilterVariant=Disabled  NVariant=Disabled  NCopyVariant=Disabled_SignalSpec  FilterICVariant=Disabled  IntegratorICVariant=InternalICs  ExternalResetVariant=Disabled  TRSumVariant=Passthrough  SumFdbkVariant=Disabled  SumVariant=Sum_PI  TsampFilterVariant=InternalTs  TsampNgainVariant=Passthrough  TsampIntegralVariant=Passthrough  ExternalSaturationOutDataTypeStr=Inherit: Same as second input  aMode=0
  Product4 : Product
  Product5 : Product
  SinCos : Trigonometry  Operator=sincos
  Omega : Outport
  theta : Outport  Port=2
  wires:
  Product4/1 -> Add8/1
  Ealpha/1 -> Product4/1
  PID Controller/1 -> Discrete-Time Integrator/1, Omega/1  "Omega"
  Discrete-Time Integrator/1 -> SinCos/1, theta/1  "theta"
  Ebeta/1 -> Product5/1
  Product5/1 -> Add8/2
  SinCos/1 -> Product5/2
  SinCos/2 -> Product4/2
  Add8/1 -> PID Controller/1  "Omega"

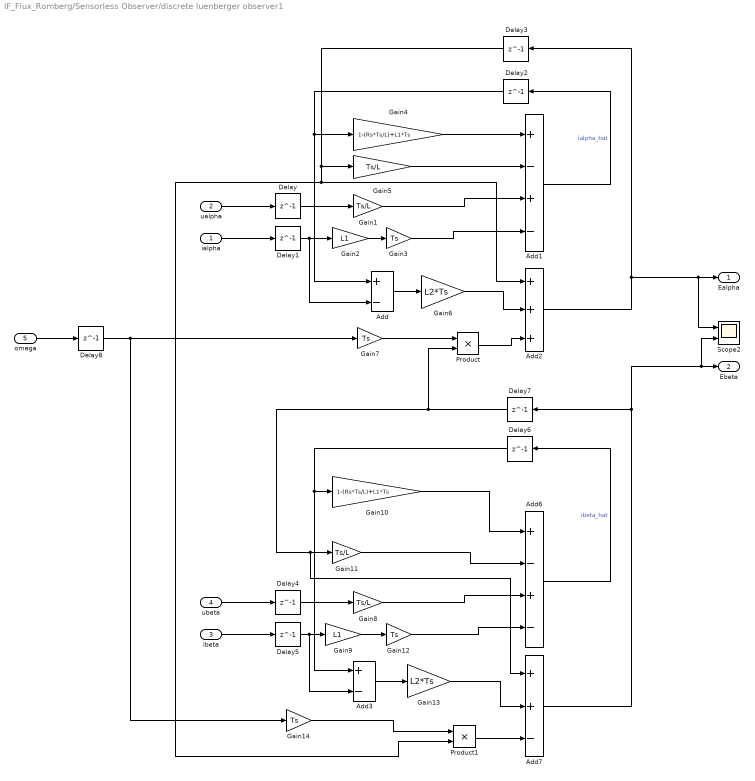
== system IF_Flux_Romberg/Sensorless Observer/discrete luenberger observer1 ==
  ialpha : Inport  OutDataTypeStr=single
  ualpha : Inport  Port=2  OutDataTypeStr=single
  ibeta : Inport  Port=3  OutDataTypeStr=single
  ubeta : Inport  Port=4  OutDataTypeStr=single
  omega : Inport  Port=5  OutDataTypeStr=single
  Add : Sum  Inputs=+-
  Add1 : Sum  Inputs=+-+-
  Add2 : Sum  Inputs=+++
  Add3 : Sum  Inputs=+-
  Add6 : Sum  Inputs=+-+-
  Add7 : Sum  Inputs=++-
  Delay{,1..8} (9 alike) : Delay  DelayLength=1
  Gain{1,5,8,11} (4 alike) : Gain  Gain=Ts/L
  Gain10 : Gain  Gain=1-(Rs*Ts/L)+L1*Ts
  Gain12 : Gain  Gain=Ts
  Gain13 : Gain  Gain=L2*Ts  OutDataTypeStr=single
  Gain14 : Gain  Gain=Ts  OutDataTypeStr=single
  Gain2 : Gain  Gain=L1
  Gain3 : Gain  Gain=Ts
  Gain4 : Gain  Gain=1-(Rs*Ts/L)+L1*Ts
  Gain6 : Gain  Gain=L2*Ts
  Gain7 : Gain  Gain=Ts
  Gain9 : Gain  Gain=L1
  Product : Product  OutDataTypeStr=single
  Product1 : Product  OutDataTypeStr=single
  Scope2 : Scope  NumInputPorts=2
  Ealpha : Outport
  Ebeta : Outport  Port=2
  wires:
  Delay8/1 -> Gain7/1, Gain14/1
  Add2/1 -> Delay3/1, Ealpha/1, Scope2/1
  ualpha/1 -> Delay/1
  ubeta/1 -> Delay4/1
  ialpha/1 -> Delay1/1
  ibeta/1 -> Delay5/1
  omega/1 -> Delay8/1
  Add7/1 -> Delay7/1, Scope2/2, Ebeta/1
  Gain10/1 -> Add6/1
  Gain8/1 -> Add6/3
  Delay4/1 -> Gain8/1
  Gain9/1 -> Gain12/1
  Delay5/1 -> Add3/2, Gain9/1
  Gain11/1 -> Add6/2
  Delay7/1 -> Add7/1, Gain11/1, Product/2
  Delay6/1 -> Add3/1, Gain10/1
  Gain14/1 -> Product1/1
  Delay3/1 -> Gain5/1, Add2/1, Product1/2
  Add6/1 -> Delay6/1  "ibeta_hat"
  Gain13/1 -> Add7/2
  Add3/1 -> Gain13/1
  Product1/1 -> Add7/3
  Gain12/1 -> Add6/4
  Add/1 -> Gain6/1
  Gain2/1 -> Gain3/1
  Gain6/1 -> Add2/2
  Gain1/1 -> Add1/3
  Delay/1 -> Gain1/1
  Delay2/1 -> Gain4/1, Add/1
  Add1/1 -> Delay2/1  "ialpha_hat"
  Gain3/1 -> Add1/4
  Product/1 -> Add2/3
  Delay1/1 -> Gain2/1, Add/2
  Gain7/1 -> Product/1
  Gain4/1 -> Add1/1
  Gain5/1 -> Add1/2

== matlab function IF_Flux_Romberg/Clark2 ==
  data: ia input; ialpha output; ib input; ic input; ibeta output
function [ialpha,ibeta] = fcn(ia,ib,ic)
ialpha = ia*2/3-(ib+ic)/3;
ibeta = (ib-ic)*sqrt(3)/3;

== matlab function IF_Flux_Romberg/Park2 ==
  data: ialpha input; ibeta input; theta input; id output; iq output
function [id,iq] = fcn(ialpha,ibeta,theta)
id = ialpha*cos(theta)+ibeta*sin(theta);
iq = -ialpha*sin(theta)+ibeta*cos(theta);

== matlab function IF_Flux_Romberg/foc1 ==
  data: ud input; Tcmp1 output; uq input; theta input; Udc input; Tpwm input; Tcmp2 output; Tcmp3 output; sector output; ts output; Valpha output; Vbeta output
function [Tcmp1,Tcmp2,Tcmp3,sector,ts,Valpha,Vbeta] = fcn(ud,uq,theta,Udc,Tpwm)

us=ud^2+uq^2;
um=(Udc^2)/3;
ud_abs=abs(ud);
beta=atan(uq/ud_abs);
if(us>um)
    ud=-sqrt(um)*cos(beta);
    uq=sqrt(um)*sin(beta);
    if(ud>0)
        ud=sqrt(um)*cos(beta);
    end
end

Valpha = ud*cos(theta) - uq*sin(theta);
Vbeta = ud*sin(theta) + uq*cos(theta);



%#codegen

sector = single(0);
Tcmp1 = single(0);
Tcmp2 = single(0);
Tcmp3 = single(0);

%========Parameters statement================

    Vref1 = Vbeta;							                   
    Vref2 = (sqrt(3)*Valpha - Vbeta)/2; 				    
    Vref3 = (-sqrt(3)*Valpha - Vbeta)/2;					
   
 %========Sector calculation=================

  if (Vref1>0)
	   sector = single(1);
  end
  if (Vref2>0)
	   sector = sector+single(2);
  end
  if (Vref3>0)
       sector = sector+single(4);
  end

%======== X Y Z calculation===================

X = sqrt(3)*Vbeta*Tpwm/Udc;
Y = Tpwm/Udc*(3/2*Valpha+sqrt(3)/2*Vbeta);
Z = Tpwm/Udc*(-3/2*Valpha+sqrt(3)/2*Vbeta);	         

%==========Duty ratio calculation================
switch (sector)   
    case 1
        T1 = Z; T2 = Y; 
	case 2
        T1 = Y; T2 = -X; 
	case 3
        T1 = -Z; T2 = X; 
	case 4
        T1 = -X; T2 = Z;
	case 5
        T1 = X; T2 = -Y;
    otherwise
        T1 = -Y; T2 = -Z;
end

    ts=T1+T2;
    
%if(ts>Tpwm)
 %   T1=Tpwm*T1/ts;
 %   T2=Tpwm*T2/ts;
 %   ts=T1+T2;
%end
ta = (Tpwm-(T1+T2))/4.0;
tb = ta+T1/2;
tc = tb+T2/2;

ta=round(ta);
tb=round(tb);
tc=round(tc);
%==========Duty ratio calculation================
switch (sector)
    case 1 
        Tcmp1=tb;
        Tcmp2=ta;
        Tcmp3=tc; 
        
    case 2 
        Tcmp1=ta;
        Tcmp2=tc;
        Tcmp3=tb; 
       
    case 3 
        Tcmp1=ta;
        Tcmp2=tb;
        Tcmp3=tc; 
        
    case 4 
        Tcmp1=tc;
        Tcmp2=tb;
        Tcmp3=ta;
        
    case 5 
        Tcmp1=tc;
        Tcmp2=ta;
        Tcmp3=tb;
        
   case 6
       Tcmp1=tb;
       Tcmp2=tc;
       Tcmp3=ta;
end
end
